simulink model "motor_model"  (R2022b)
settings: Solver=VariableStepAuto  StartTime=0.0  StopTime=10.0  RelTol=1e-3
settings Model: Creator=User  LastModifiedBy=User

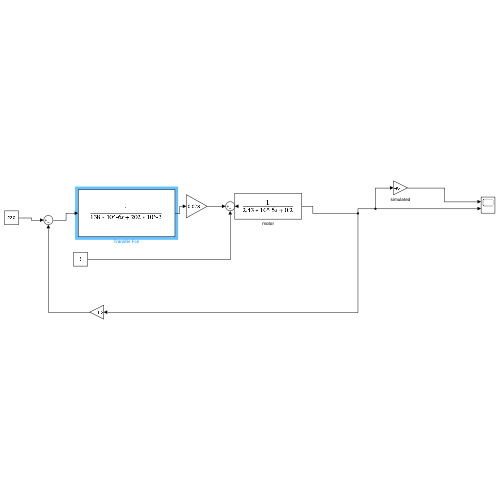
[thumbnail: Simulink's stored preview of the top-level diagram]
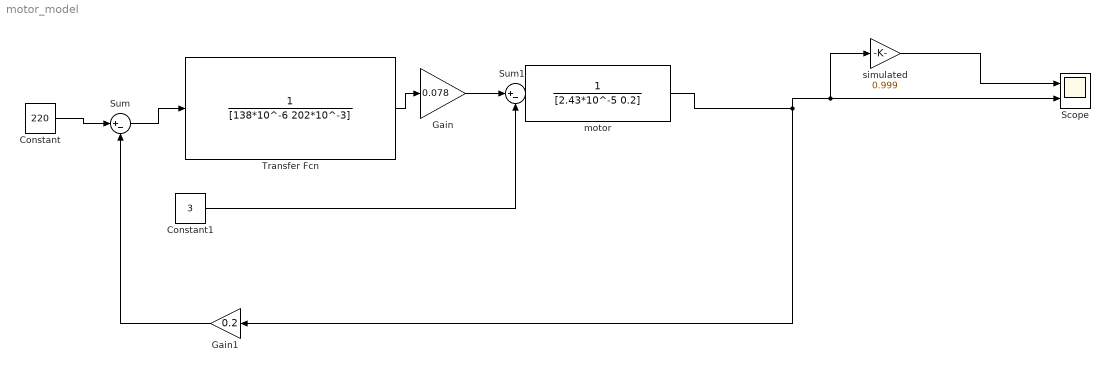
== system motor_model ==
  Constant : Constant  Value=220
  Constant1 : Constant  Value=3
  Gain : Gain  Gain=0.078
  Gain1 : Gain  Gain=0.2
  Scope : Scope  NumInputPorts=2
  Sum : Sum  Inputs=|+-
  Sum1 : Sum  Inputs=|+-
  Transfer Fcn : TransferFcn  Denominator=[138*10^-6 202*10^-3]
  motor : TransferFcn  Denominator=[2.43*10^-5 0.2]
  simulated : Gain  Gain=0.999
  wires:
  Sum/1 -> Transfer Fcn/1
  Transfer Fcn/1 -> Gain/1
  Constant/1 -> Sum/1
  Gain/1 -> Sum1/1
  Constant1/1 -> Sum1/2
  Sum1/1 -> motor/1
  Gain1/1 -> Sum/2
  motor/1 -> simulated/1, Scope/2, Gain1/1
  simulated/1 -> Scope/1
